simulink model "concept3_simulink_RL"  (R2025a)
settings: Solver=VariableStepAuto  StartTime=0.0  StopTime=Tf  FixedStep=0.001  MaxStep=0.01  MinStep=0.0001  RelTol=1e-3
InitFcn:
  | loaded_data = load('concept3_for_sim.mat');
  | robot = loaded_data.robot;
  | robot.DataFormat = 'column';
values from neighbouring files (symbols this model uses):
  mass = 40    [RL_main.m]    (also in baseline_sim.m)
  obs_vec = opa    [RL_main.m]    (also in baseline_sim.m)
  port = data(n, :)    [RL_main.m]    (also in baseline_sim.m = port_pos_data(n,:))
  port_num = 10    [RL_main.m]    (also in baseline_sim.m)
  port_target = AB2port(port_num)    [RL_main.m]    (also in baseline_sim.m)
  q0arm = rad2deg([-1.283; -1.622; 2.2761853; -1.8021853; 1.112; 1.859; 0.05328])    [RL_main.m]    (also in baseline_sim.m)
  q0b = [1; 0; 0; 0; 0; 0; 0]    [RL_main.m]    (also in baseline_sim.m = [1;0;0;0;0;0;0])
  sat_docked = AB2port(sat_docked_num)    [RL_main.m]    (also in baseline_sim.m)
  sat_docked_num = 6    [RL_main.m]    (also in baseline_sim.m)
  sim_state = 1    [RL_main.m]    (also in baseline_sim.m)
  Tlog = 0.1    [RL_main.m]    (also in baseline_sim.m)
  use_RL = 1    [RL_main.m]    (also in baseline_sim.m)
undefined symbols (not defined in the file or in its folder): opa, target, X, Y, Z
libraries: sm_lib x133, nesl_utility x67, simulink_extras x3, rllib x2
(part 1 of 6)
settings Model: Creator=Junesuk  LastModifiedBy=Junesuk
settings ExplorerConfigSet: InternalSimMechanicsExplorerSettings=|
  | <ExplorerConfiguration>
  | 
  |   <canonicalview>default</canonicalview>
  | 
  |   <TilePanel>
  |     <TileInfo>
  |       <Tiles Columns="1" Count="1" Height="644" Rows="1" Width="984">
  |         <Row Weight="1"/>
  |         <Column Weight="1"/>
  |         <Tile Height="1" Width="1" X="0" Y="0"/>
  |       </Tiles>
  |     </TileInfo>
  |     <SceneInfo>
  |       <SceneViewer>
  |         <IsThisViewStd>
  |           <IsStandardView>off</IsStandardView>
  |           <StandardViewName>Front</StandardViewName>
  |         </IsThisViewStd>
  |         <BGColor>
  |           <R>1</R>
  |           <G>1</G>
  |           <B>1</B>
  |           <A>1</A>
  |         </BGColor>
  |         <Camera>
  |           <DoPerspective>off</DoPerspective>
  |           <Position>
  |             <X>21.646149636080793</X>
  |             <Y>-1.0053245677685836</Y>
  |             <Z>2.2639877275739697</Z>
  |           </Position>
  |           <Center>
  |             <X>0.33501300739641093</X>
  |             <Y>0.083525792263903942</Y>
  |             <Z>0.40625179063450656</Z>
  |           </Center>
  |           <Up>
  |             <X>-0.095945200689781199</X>
  |             <Y>-0.22258518034193089</Y>
  |             <Z>0.97018057904533828</Z>
  |           </Up>
  |           <XLim>2.365123016199409</XLim>
  |           <YLim>2.365123016199409</YLim>
  |           <ViewLimDist>0.01</ViewLimDist>
  |         </Camera>
  |       </SceneViewer>
  |     </SceneInfo>
  |   </TilePanel>
  | 
  |   <MechEditorPanel>
  |     <GfxPanelCameraMap/>
  |     <Cameras/>
  |     <VideoCreator>
  |       <IncludeTiles>All</IncludeTiles>
  |       <IncludeTime>on</IncludeTime>
  |       <IncludeWorldFrame>off</IncludeWorldFrame>
  |       <PlaybackSpeedRatio>1</PlaybackSpeedRatio>
  |       <FrameRate>30</FrameRate>
  |       <FrameSize>auto</FrameSize>
  |       <VideoFormat>UncompressedAVI</VideoFormat>
  |     </VideoCreator>
  |   </MechEditorPanel>
  | 
  |   <PlaybackSettings>
  |     <PlaybackSpeedFactor>16</PlaybackSpeedFactor>
  |   </PlaybackSettings>
  | 
  | </ExplorerConfiguration>

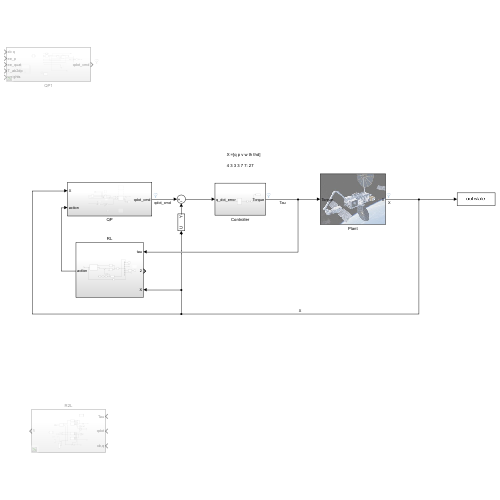
[thumbnail: Simulink's stored preview of the top-level diagram]
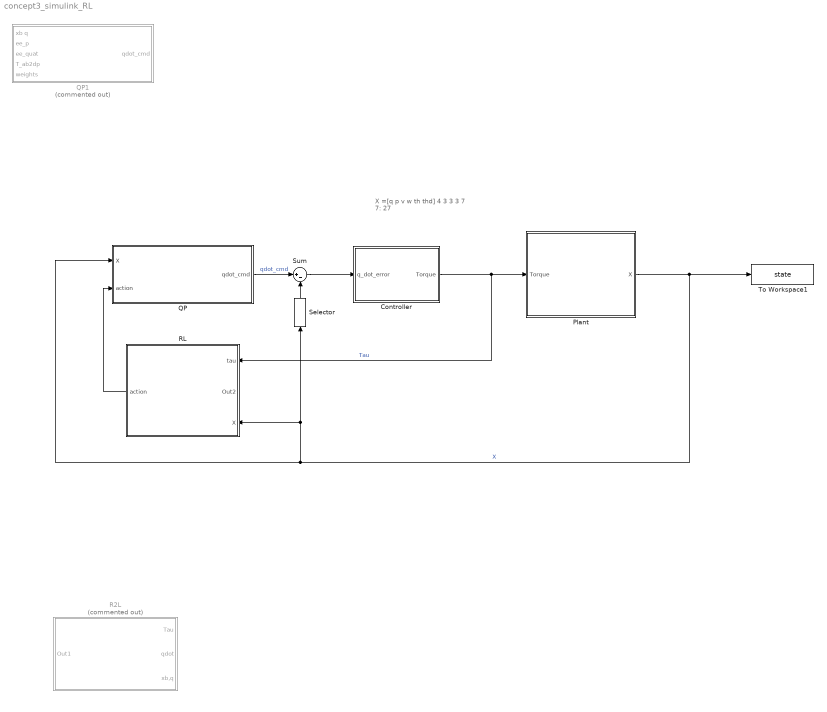
== system concept3_simulink_RL ==
  note: X =[q p v w th thd]
      |
      | 4 3 3 3 7 7: 27
  Controller : Subsystem
  Plant : Subsystem
      mask Display: image('1.jpg');
  QP : Subsystem
  QP1 : Subsystem  Commented=on
  R2L : Subsystem  Commented=on
  RL : Subsystem
      settings: PortSchema="{\"entries\":[{\"content\":{\"sides\":[{\"content\":{\"connectorIds\":[\"In1\",\"Out2\",\"In2\"]},\"type\":\"ConnectorPlacement.EquallySpacedRectSide\",\"uuid\":\"81336b0f-87da-4949-bb3f-96bdd0722e32\"},{\"content\":{\"connectorIds\":[\"Out1\"],\"side\":\"RIGHT\"},\"type\":\"ConnectorPlacement.EquallySpacedRectSide\",\"uuid\":\"5ebe1975-ec97-4e49-ac6a-50b9e3487ed2\"},{\"content\":{\"side\":\"TOP\"},\"type\":\"ConnectorPlacement.EquallySpacedRectSide\",\"uuid\":\"c24f2ad8-8f66-451d-b311-007f5efa803c\"}]},\"type\":\"ConnectorPlacement.EquallySpacedConnector\",\"uuid\":\"e8b94ec5-1840-41b7-8daf-8d62ee1595ef\"}],\"packageUris\":[\"http://schema.mathworks.com/mf0/Connector/R2020b\"],\"version\":\"1.0\"}"
  Selector : Selector  InputPortWidth=27  IndexOptions=Index vector (dialog)  Indices=[21 22 23 24 25 26 27]  OutputSizes=1
  Sum : Sum  Inputs=|+-
  To Workspace1 : ToWorkspace  VariableName=state  SaveFormat=Timeseries  SampleTime=Tlog
  wires:
  Plant/1(X) -> To Workspace1/1, QP/1(X), Selector/1, RL/2(X)  "X"
  Sum/1 -> Controller/1(q_dot_error)
  Controller/1(Torque) -> RL/1(tau), Plant/1(Torque)  "Tau"
  QP/1(qdot_cmd) -> Sum/1  "qdot_cmd"
  RL/1(action) -> QP/2(action)
  Selector/1 -> Sum/2

== system concept3_simulink_RL/Controller ==
  q_dot_error : Inport
  MATLAB Function : MATLAB Function  TreatAsAtomicUnit=on
  Rate Limiter : RateLimiter  RisingSlewLimit=80  FallingSlewLimit=-80  SampleTimeMode=inherited
  Saturation : Saturate  UpperLimit=3  LowerLimit=-3
  To Workspace1 : ToWorkspace  VariableName=torque  SaveFormat=Timeseries  SampleTime=Tlog
  Torque : Outport
  wires:
  Saturation/1 -> To Workspace1/1, Torque/1
  q_dot_error/1 -> MATLAB Function/1(qdot_err)
  MATLAB Function/1(Torque) -> Rate Limiter/1
  Rate Limiter/1 -> Saturation/1

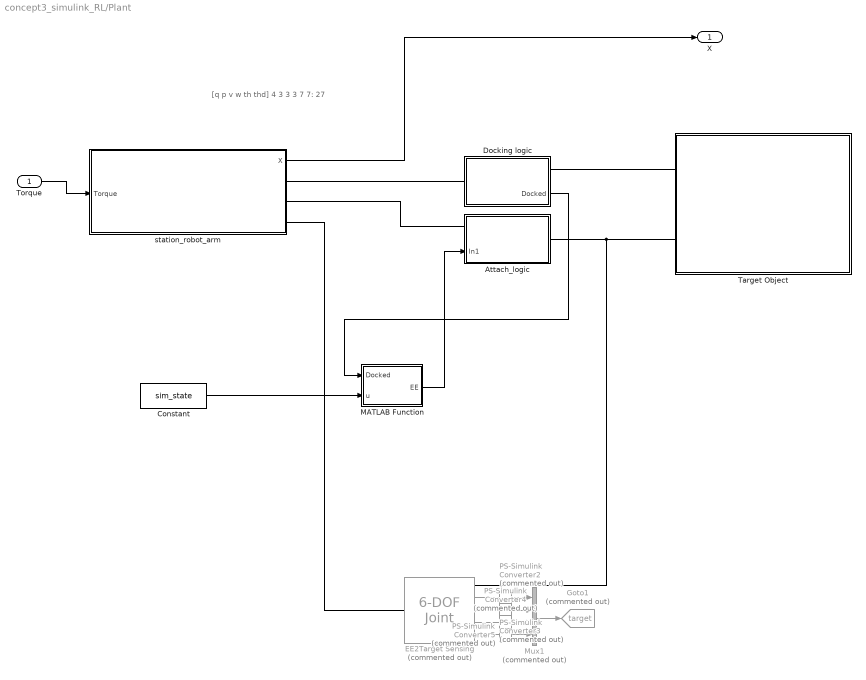
== system concept3_simulink_RL/Plant ==
  note: [q p v w th thd]
      |
      | 4 3 3 3 7 7: 27
  Torque : Inport
  Attach_logic : Subsystem
      settings: PortSchema="{\"entries\":[{\"content\":{\"sides\":[{\"content\":{\"connectorIds\":[\"LConn1\",\"In1\"]},\"type\":\"ConnectorPlacement.EquallySpacedRectSide\",\"uuid\":\"12d0cedd-e218-4f17-9320-f216ac9747ac\"},{\"content\":{\"connectorIds\":[\"RConn1\"],\"side\":\"RIGHT\"},\"type\":\"ConnectorPlacement.EquallySpacedRectSide\",\"uuid\":\"fd28970a-cca5-4053-a7a0-12fc7f529469\"},{\"content\":{\"side\":\"TOP\"},\"type\":\"ConnectorPlacement.EquallySpacedRectSide\",\"uuid\":\"e9d689cc-5bb9-4a0d-a40b-d0a8c8edca38\"}]},\"type\":\"ConnectorPlacement.EquallySpacedConnector\",\"uuid\":\"9791f5c1-0484-4ef0-8b6a-77682d20579a\"}],\"packageUris\":[\"http://schema.mathworks.com/mf0/Connector/R2020b\"],\"version\":\"1.0\"}"
  Constant : Constant  Value=sim_state
  Docking logic : Subsystem
      settings: PortSchema="{\"entries\":[{\"content\":{\"sides\":[{\"content\":{\"connectorIds\":[\"LConn1\"]},\"type\":\"ConnectorPlacement.EquallySpacedRectSide\",\"uuid\":\"76e864fd-fcf6-40cb-8d0c-a293f5f8e793\"},{\"content\":{\"connectorIds\":[\"RConn1\",\"Out1\"],\"side\":\"RIGHT\"},\"type\":\"ConnectorPlacement.EquallySpacedRectSide\",\"uuid\":\"51e0a38e-4dda-40d7-8539-b3b2212d4dbb\"},{\"content\":{\"side\":\"TOP\"},\"type\":\"ConnectorPlacement.EquallySpacedRectSide\",\"uuid\":\"08ea25f5-31f4-4a06-bacf-9e22bf3b7d63\"}]},\"type\":\"ConnectorPlacement.EquallySpacedConnector\",\"uuid\":\"c97bdcdc-89c7-4c9e-882d-350e4fa10246\"}],\"packageUris\":[\"http://schema.mathworks.com/mf0/Connector/R2020b\"],\"version\":\"1.0\"}"
  EE2Target Sensing : sm_lib/Joints/6-DOF Joint  Commented=on  JointMode=Normal  CompositeWrenchDir=FollowerOnBase  CompositeWrenchFrame=BaseFrame  SenseConstraintForce=off  SenseConstraintTorque=off  SenseTotalForce=off  SenseTotalTorque=off  PxPositionTargetSpecify=on  PxPositionTargetPriority=Low  PxPositionTargetValue=target(1)  PxPositionTargetValueUnits=m  PxVelocityTargetSpecify=off  PxVelocityTargetPriority=High  PxVelocityTargetValue=0  PxVelocityTargetValueUnits=m/s  PxEquilibriumPosition=0  PxEquilibriumPositionUnits=m  PxSpringStiffness=0  PxSpringStiffnessUnits=N/m  PxDampingCoefficient=0  PxDampingCoefficientUnits=N/(m/s)  PxLowerLimitSpecify=off  PxLowerLimitBound=-1  PxLowerLimitBoundUnits=m  PxLowerLimitStiffness=1e6  PxLowerLimitStiffnessUnits=N/m  PxLowerLimitDamping=1e3  PxLowerLimitDampingUnits=N/(m/s)  PxLowerLimitTransitionRegionWidth=1e-4  PxLowerLimitTransitionRegionWidthUnits=m  PxUpperLimitSpecify=off  PxUpperLimitBound=1  PxUpperLimitBoundUnits=m  PxUpperLimitStiffness=1e6  PxUpperLimitStiffnessUnits=N/m  PxUpperLimitDamping=1e3  PxUpperLimitDampingUnits=N/(m/s)  PxUpperLimitTransitionRegionWidth=1e-4  PxUpperLimitTransitionRegionWidthUnits=m  PxTorqueActuationMode=NoTorque  PxMotionActuationMode=ComputedMotion  PxSensePosition=on  PxSenseVelocity=off  PxSenseAcceleration=off  PxSenseTorqueForce=off  PxSenseLowerLimitTorqueForce=off  PxSenseUpperLimitTorqueForce=off  PyPositionTargetSpecify=on  PyPositionTargetPriority=Low  PyPositionTargetValue=target(2)  PyPositionTargetValueUnits=m  PyVelocityTargetSpecify=off  PyVelocityTargetPriority=High  PyVelocityTargetValue=0  PyVelocityTargetValueUnits=m/s  PyEquilibriumPosition=0  PyEquilibriumPositionUnits=m  PySpringStiffness=0  PySpringStiffnessUnits=N/m  PyDampingCoefficient=0  PyDampingCoefficientUnits=N/(m/s)  PyLowerLimitSpecify=off  PyLowerLimitBound=-1  PyLowerLimitBoundUnits=m  PyLowerLimitStiffness=1e6  PyLowerLimitStiffnessUnits=N/m  PyLowerLimitDamping=1e3  PyLowerLimitDampingUnits=N/(m/s)  PyLowerLimitTransitionRegionWidth=1e-4  PyLowerLimitTransitionRegionWidthUnits=m  PyUpperLimitSpecify=off  PyUpperLimitBound=1  PyUpperLimitBoundUnits=m  PyUpperLimitStiffness=1e6  PyUpperLimitStiffnessUnits=N/m  PyUpperLimitDamping=1e3  PyUpperLimitDampingUnits=N/(m/s)  PyUpperLimitTransitionRegionWidth=1e-4  PyUpperLimitTransitionRegionWidthUnits=m  PyTorqueActuationMode=NoTorque  PyMotionActuationMode=ComputedMotion  PySensePosition=on  PySenseVelocity=off  PySenseAcceleration=off  PySenseTorqueForce=off  PySenseLowerLimitTorqueForce=off  PySenseUpperLimitTorqueForce=off  PzPositionTargetSpecify=on  PzPositionTargetPriority=Low  PzPositionTargetValue=target(3)  PzPositionTargetValueUnits=m  PzVelocityTargetSpecify=off  PzVelocityTargetPriority=High  PzVelocityTargetValue=0  PzVelocityTargetValueUnits=m/s  PzEquilibriumPosition=0  PzEquilibriumPositionUnits=m  PzSpringStiffness=0  PzSpringStiffnessUnits=N/m  PzDampingCoefficient=0  PzDampingCoefficientUnits=N/(m/s)  PzLowerLimitSpecify=off  PzLowerLimitBound=-1  PzLowerLimitBoundUnits=m  PzLowerLimitStiffness=1e6  PzLowerLimitStiffnessUnits=N/m  PzLowerLimitDamping=1e3  PzLowerLimitDampingUnits=N/(m/s)  PzLowerLimitTransitionRegionWidth=1e-4  PzLowerLimitTransitionRegionWidthUnits=m  PzUpperLimitSpecify=off  PzUpperLimitBound=1  PzUpperLimitBoundUnits=m  PzUpperLimitStiffness=1e6  PzUpperLimitStiffnessUnits=N/m  PzUpperLimitDamping=1e3  PzUpperLimitDampingUnits=N/(m/s)  PzUpperLimitTransitionRegionWidth=1e-4  PzUpperLimitTransitionRegionWidthUnits=m  PzTorqueActuationMode=NoTorque  PzMotionActuationMode=ComputedMotion  PzSensePosition=on  PzSenseVelocity=off  PzSenseAcceleration=off  PzSenseTorqueForce=off  PzSenseLowerLimitTorqueForce=off  PzSenseUpperLimitTorqueForce=off  SphPositionTargetSpecify=on  SphPositionTargetPriority=Low  SphPositionTargetRotationMethod=RotationSequence  SphPositionTargetFollAlignAxisA=+X  SphPositionTargetBaseAlignAxisA=+Y  SphPositionTargetFollAlignAxisB=+Y  SphPositionTargetBaseAlignAxisB=+Z  SphPositionTargetRotationStandardAxis=+Z  SphPositionTargetRotationAngle=0  SphPositionTargetRotationAngleUnits=deg  SphPositionTargetRotationArbitraryAxis=[0 0 1]  SphPositionTargetRotationSequenceAxes=FollowerAxes  SphPositionTargetRotationSequence=ZYX  SphPositionTargetRotationSequenceAngles=[target(4) target(5) target(6) ]  SphPositionTargetRotationSequenceAnglesUnits=deg  SphPositionTargetRotationMatrix=[1 0 0;0 1 0;0 0 1]  SphPositionTargetQuaternion=[1 0 0 0]  SphVelocityTargetSpecify=off  SphVelocityTargetPriority=High  SphVelocityTargetValue=[0 0 0]  SphVelocityTargetValueUnits=deg/s  SphVelocityTargetInFollowerFrame=on  SphEqPosRotationMethod=None  SphEqPosFollAlignAxisA=+X  SphEqPosBaseAlignAxisA=+Y  SphEqPosFollAlignAxisB=+Y  SphEqPosBaseAlignAxisB=+Z  SphEqPosRotationStandardAxis=+Z  SphEqPosRotationAngle=0  SphEqPosRotationAngleUnits=deg  SphEqPosRotationArbitraryAxis=[0 0 1]  SphEqPosRotationSequenceAxes=FollowerAxes  SphEqPosRotationSequence=XYX  SphEqPosRotationSequenceAngles=[0 0 0]  SphEqPosRotationSequenceAnglesUnits=deg  SphEqPosRotationMatrix=[1 0 0;0 1 0;0 0 1]  SphEqPosQuaternion=[1 0 0 0]  SphSpringStiffness=0  SphSpringStiffnessUnits=N*m/deg  SphDampingCoefficient=0  SphDampingCoefficientUnits=N*m/(deg/s)  SphLowerLimitSpecify=off  SphLowerLimitBound=15  SphLowerLimitBoundUnits=deg  SphLowerLimitStiffness=1e4  SphLowerLimitStiffnessUnits=N*m/deg  SphLowerLimitDamping=10  SphLowerLimitDampingUnits=N*m/(deg/s)  SphLowerLimitTransitionRegionWidth=0.1  SphLowerLimitTransitionRegionWidthUnits=deg  SphUpperLimitSpecify=off  SphUpperLimitBound=45  SphUpperLimitBoundUnits=deg  SphUpperLimitStiffness=1e4  SphUpperLimitStiffnessUnits=N*m/deg  SphUpperLimitDamping=10  SphUpperLimitDampingUnits=N*m/(deg/s)  SphUpperLimitTransitionRegionWidth=0.1  SphUpperLimitTransitionRegionWidthUnits=deg  SphTorqueActuationMode=NoTorque  SphActuateTorqueX=off  SphActuateTorqueY=off  SphActuateTorqueZ=off  SphActuateTorque=off  SphActuationFrame=BaseFrame  SphSensePosition=on  SphSenseVelocityX=off  SphSenseVelocityY=off  SphSenseVelocityZ=off  SphSenseVelocity=off  SphSenseAccelerationX=off  SphSenseAccelerationY=off  SphSenseAccelerationZ=off  SphSenseAcceleration=off  SphSenseLowerLimitTorqueMag=off  SphSenseUpperLimitTorqueMag=off  SphSensingFrame=BaseFrame
  Goto1 : Goto  Commented=on  GotoTag=target  TagVisibility=global
  MATLAB Function : MATLAB Function  TreatAsAtomicUnit=on
  Mux1 : Mux  Commented=on
  PS-Simulink Converter{2..5} (4 alike) : nesl_utility/PS-Simulink Converter  Commented=on  PhysicalDomain=network_engine_domain  SubClassName=ps_output  LeftPortType=input  RightPortType=output  PseudoPeriodic=off  Frequencies=[]  VectorFormat=inherit  Unit=inherit  AffineConversion=off
  Target Object : Subsystem
      mask Display: image('2.jpg');
  station_robot_arm : Subsystem
  X : Outport
  wires:
  Torque/1 -> station_robot_arm/1(Torque)
  station_robot_arm/1(X) -> X/1
  PS-Simulink Converter2/1 -> Mux1/1
  PS-Simulink Converter3/1 -> Mux1/2
  PS-Simulink Converter4/1 -> Mux1/3
  PS-Simulink Converter5/1 -> Mux1/4
  Mux1/1 -> Goto1/1
  Constant/1 -> MATLAB Function/2(u)
  MATLAB Function/1(EE) -> Attach_logic/1(In1)
  Docking logic/1(Docked) -> MATLAB Function/1(Docked)
  connections:
  Target Object/LConn1 -- Docking logic/RConn1
  Attach_logic/RConn1 -- EE2Target Sensing/RConn1 -- Target Object/LConn2
  station_robot_arm/RConn3 -- EE2Target Sensing/LConn1
  station_robot_arm/RConn2 -- Attach_logic/LConn1
  station_robot_arm/RConn1 -- Docking logic/LConn1
  PS-Simulink Converter4/LConn1 -- EE2Target Sensing/RConn4
  EE2Target Sensing/RConn3 -- PS-Simulink Converter3/LConn1
  EE2Target Sensing/RConn2 -- PS-Simulink Converter2/LConn1
  PS-Simulink Converter5/LConn1 -- EE2Target Sensing/RConn5

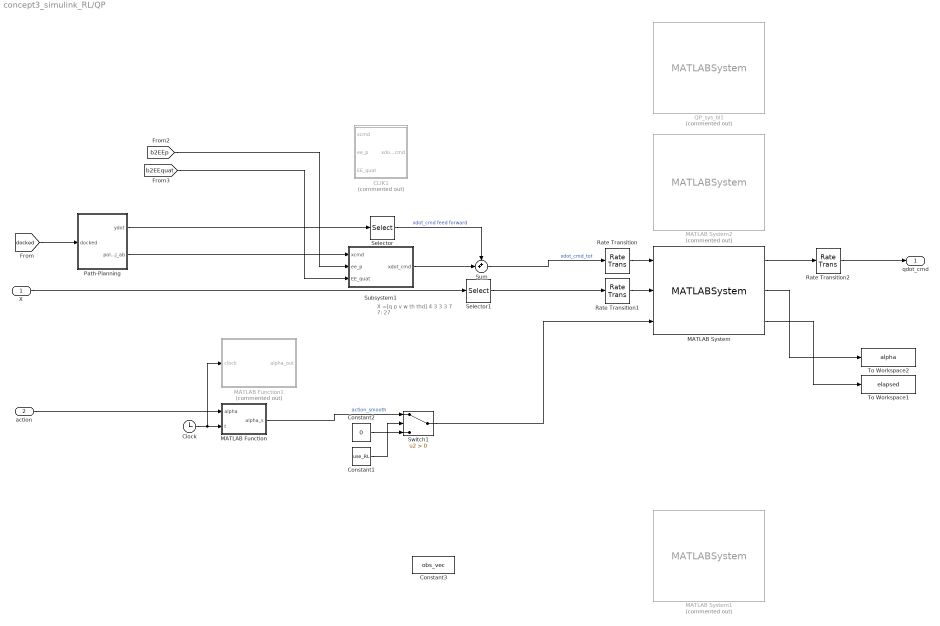
== system concept3_simulink_RL/QP ==
  note: X =[q p v w th thd]
      |
      | 4 3 3 3 7 7: 27
  X : Inport
  action : Inport  Port=2
  CLIK1 : Subsystem  Commented=on
  Clock : Clock
  Constant1 : Constant  Value=use_RL
  Constant2 : Constant  Value=0
  Constant3 : Constant  Value=obs_vec
  MATLAB Function : MATLAB Function  TreatAsAtomicUnit=on
  MATLAB Function1 : MATLAB Function  Commented=on  TreatAsAtomicUnit=on
  MATLAB System : MATLABSystem  System=QP_sys_RL  SimulateUsing=Interpreted execution
      mask Type: QP_sys_RL
  MATLAB System1 : MATLABSystem  Commented=on  System=RH_QP_sys_bl  H_hor=10  lambda_s=0.05  lambda_t=0.1  kp_base=10  SimulateUsing=Interpreted execution
      mask Type: RH_QP_sys_bl
  MATLAB System2 : MATLABSystem  Commented=on  System=Pseudo_inv_sys_RL  SimulateUsing=Interpreted execution
      mask Type: Pseudo_inv_sys_RL
  "Path-Planning " : Subsystem
  QP_sys_bl1 : MATLABSystem  Commented=on  System=QP_sys_bl  null_method=a  kp_base=1  SimulateUsing=Interpreted execution
      mask Type: QP_sys_bl
  Rate Transition : RateTransition  OutPortSampleTime=Tq
  Rate Transition1 : RateTransition  OutPortSampleTime=Tq
  Rate Transition2 : RateTransition
  Selector : Selector  InputPortWidth=6  IndexOptions=Index vector (dialog)  Indices=[4 5 6 1 2 3]  OutputSizes=1
  Selector1 : Selector  InputPortWidth=27  IndexOptions=Index vector (dialog)  Indices=[1 2 3 4 5 6 7 14 15 16 17 18 19 20]  OutputSizes=1
  Subsystem1 : Subsystem
  Sum : Sum  Inputs=++|
  Switch1 : Switch  Criteria=u2 > Threshold  SaturateOnIntegerOverflow=off  InputSameDT=off
  To Workspace1 : ToWorkspace  VariableName=elapsed  SaveFormat=Timeseries  SampleTime=Tlog
  To Workspace2 : ToWorkspace  VariableName=alpha  SaveFormat=Timeseries  SampleTime=Tlog
  qdot_cmd : Outport
  wires:
  [docked] -> "Path-Planning "/1(docked)
  "Path-Planning "/1(ydot) -> Selector/1
  "Path-Planning "/2(poly_traj_ab) -> Subsystem1/1(xcmd)
  Subsystem1/1(xdot_cmd) -> Sum/2
  [b2EEp] -> Subsystem1/2(ee_p)
  [b2EEquat] -> Subsystem1/3(EE_quat)
  Sum/1 -> Rate Transition/1  "xdot_cmd_tot"
  Clock/1 -> MATLAB Function1/1(clock), MATLAB Function/2(t)
  Constant2/1 -> Switch1/3
  MATLAB Function/1(alpha_s) -> Switch1/1  "action_smooth"
  X/1 -> Selector1/1
  Selector1/1 -> Rate Transition1/1
  Rate Transition/1 -> MATLAB System/1
  Rate Transition2/1 -> qdot_cmd/1
  Constant1/1 -> Switch1/2
  action/1 -> MATLAB Function/1(alpha)
  Selector/1 -> Sum/1  "xdot_cmd feed forward"
  MATLAB System/1 -> Rate Transition2/1
  MATLAB System/3 -> To Workspace1/1
  Rate Transition1/1 -> MATLAB System/2
  MATLAB System/2 -> To Workspace2/1
  Switch1/1 -> MATLAB System/3

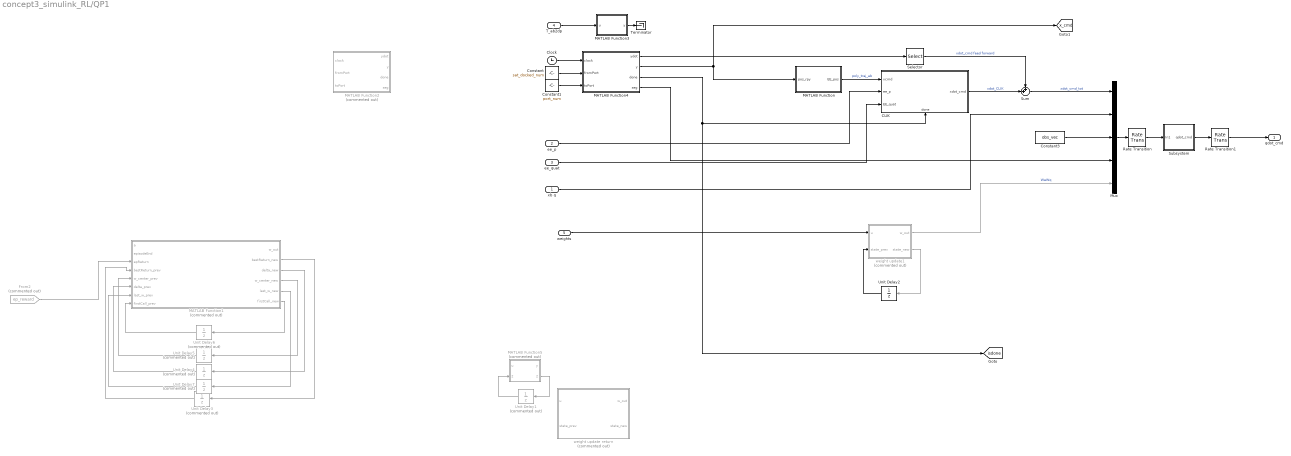
== system concept3_simulink_RL/QP1 ==
  xb q : Inport
  ee_p : Inport  Port=2
  ee_quat : Inport  Port=3
  T_ab2dp : Inport  Port=4
  weights : Inport  Port=5
  CLIK : Subsystem
      settings: PortSchema="{\"entries\":[{\"content\":{\"sides\":[{\"content\":{\"connectorIds\":[\"In1\",\"In2\",\"In3\"]},\"type\":\"ConnectorPlacement.EquallySpacedRectSide\",\"uuid\":\"53537e45-b349-4ff7-b811-6fdcc057d7d2\"},{\"content\":{\"connectorIds\":[\"Out1\"],\"side\":\"RIGHT\"},\"type\":\"ConnectorPlacement.EquallySpacedRectSide\",\"uuid\":\"c6f0bded-37ff-429d-8334-4fbe19a63c08\"},{\"content\":{\"side\":\"TOP\"},\"type\":\"ConnectorPlacement.EquallySpacedRectSide\",\"uuid\":\"dac46d9f-48be-42ca-88ab-9eef949b6b0e\"},{\"content\":{\"connectorIds\":[\"In4\"],\"side\":\"BOTTOM\"},\"type\":\"ConnectorPlacement.EquallySpacedRectSide\",\"uuid\":\"26bd092c-8c32-427f-a0d8-6b9ca2752a43\"}]},\"type\":\"ConnectorPlacement.EquallySpacedConnector\",\"uuid\":\"0be7ea49-038f-4080-8c33-dbecb36af2ab\"}],\"packageUris\":[\"http://schema.mathworks.com/mf0/Connector/R2020b\"],\"version\":\"1.0\"}"
  Clock : Clock
  Constant : Constant  Value=sat_docked_num
  Constant1 : Constant  Value=port_num
  Constant3 : Constant  Value=obs_vec
  From2 : From  Commented=on  GotoTag=ep_reward  TagVisibility=global
  MATLAB Function : MATLAB Function  TreatAsAtomicUnit=on
  MATLAB Function1 : MATLAB Function  Commented=on  TreatAsAtomicUnit=on
  MATLAB Function2 : MATLAB Function  Commented=on  TreatAsAtomicUnit=on
  MATLAB Function3 : MATLAB Function  TreatAsAtomicUnit=on
  MATLAB Function4 : MATLAB Function  TreatAsAtomicUnit=on
  MATLAB Function5 : MATLAB Function  Commented=on  TreatAsAtomicUnit=on
  Mux : Mux  Inputs=5
  Rate Transition : RateTransition  OutPortSampleTime=0.1
  Rate Transition1 : RateTransition
  Selector : Selector  InputPortWidth=6  IndexOptions=Index vector (dialog)  Indices=[4 5 6 1 2 3]  OutputSizes=1
  Subsystem : Subsystem
  Sum : Sum  Inputs=++|
  Terminator : Terminator
  Unit Delay{1,3..7} (6 alike) : UnitDelay  Commented=on  SampleTime=-1  HasFrameUpgradeWarning=on
  Unit Delay2 : UnitDelay  SampleTime=-1  HasFrameUpgradeWarning=on
  weight update return : MATLAB Function  Commented=on  TreatAsAtomicUnit=on
  weight update1 : MATLAB Function  Commented=on  TreatAsAtomicUnit=on
  qdot_cmd : Outport
  tag scope: isdone=global, x_cmd=global
  wires:
  MATLAB Function4/3(done) -> CLIK/4(done), [isdone]
  MATLAB Function3/1(y) -> Terminator/1
  Unit Delay6/1 -> MATLAB Function1/8(firstCall_prev)
  MATLAB Function1/6(firstCall_new) -> Unit Delay6/1
  Unit Delay7/1 -> MATLAB Function1/7(last_w_prev)
  MATLAB Function1/5(last_w_new) -> Unit Delay7/1
  Unit Delay4/1 -> MATLAB Function1/6(delta_prev)
  MATLAB Function1/3(delta_new) -> Unit Delay4/1
  Unit Delay5/1 -> MATLAB Function1/5(w_center_prev)
  MATLAB Function1/4(w_center_new) -> Unit Delay5/1
  Unit Delay3/1 -> MATLAB Function1/4(bestReturn_prev)
  MATLAB Function1/2(bestReturn_new) -> Unit Delay3/1
  weights/1 -> weight update1/1(u)
  Unit Delay2/1 -> weight update1/2(state_prev)
  weight update1/2(state_new) -> Unit Delay2/1
  From2/1 -> MATLAB Function1/3(epReturn)
  weight update1/1(w_out) -> Mux/5  "WeWq"
  Unit Delay1/1 -> MATLAB Function5/2(w_prev)
  MATLAB Function5/2(w_new) -> Unit Delay1/1
  Rate Transition1/1 -> qdot_cmd/1
  Rate Transition/1 -> Subsystem/1(In1)
  Mux/1 -> Rate Transition/1
  Subsystem/1(qdot_cmd) -> Rate Transition1/1
  MATLAB Function4/4(seg) -> Mux/4
  CLIK/1(xdot_cmd) -> Sum/2  "xdot_CLIK"
  Constant3/1 -> Mux/3
  T_ab2dp/1 -> MATLAB Function3/1(u)
  MATLAB Function4/2(y) -> MATLAB Function/1(pos_rpy), [x_cmd]
  MATLAB Function4/1(ydot) -> Selector/1
  Selector/1 -> Sum/1  "xdot_cmd feed forward"
  Sum/1 -> Mux/1  "xdot_cmd_tot"
  MATLAB Function/1(EE_pos) -> CLIK/1(xcmd)  "poly_traj_ab"
  ee_quat/1 -> CLIK/3(EE_quat)
  ee_p/1 -> CLIK/2(ee_p)
  Constant1/1 -> MATLAB Function4/3(toPort)
  Constant/1 -> MATLAB Function4/2(fromPort)
  Clock/1 -> MATLAB Function4/1(clock)
  xb q/1 -> Mux/2

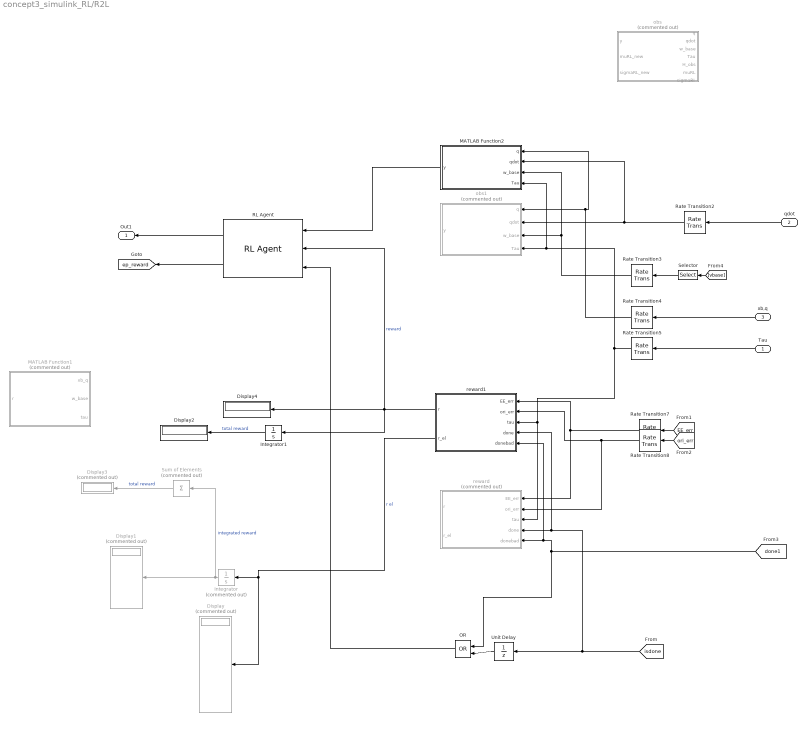
== system concept3_simulink_RL/R2L ==
  Tau : Inport
  qdot : Inport  Port=2
  xb,q : Inport  Port=3
  Display : Display  Commented=on
  Display1 : Display  Commented=on
  Display2 : Display
  Display3 : Display  Commented=on
  Display4 : Display
  Integrator : Integrator  Commented=on
  Integrator1 : Integrator
  MATLAB Function1 : MATLAB Function  Commented=on  TreatAsAtomicUnit=on
  MATLAB Function2 : MATLAB Function  TreatAsAtomicUnit=on
  OR : Logic  Operator=OR  IconShape=distinctive  AllPortsSameDT=off  OutDataTypeStr=boolean
  RL Agent : rllib/RL Agent  Agent=agent  ExternalActionAsInput=off  ProvideLastAction=off  ProvideCumRwd=on  TreatAsDirectFeedthrough=on  UseStrictObservationDataTypes=off
  Rate Transition{2..5,7..8} (6 alike) : RateTransition  OutPortSampleTime=Ts
  Selector : Selector  InputPortWidth=6  IndexOptions=Index vector (dialog)  Indices=[4 5 6]  OutputSizes=1
  Sum of Elements : Sum  Commented=on  Inputs=+
  Unit Delay : UnitDelay  SampleTime=-1  HasFrameUpgradeWarning=on
  obs : MATLAB Function  Commented=on  TreatAsAtomicUnit=on
  obs1 : MATLAB Function  Commented=on  TreatAsAtomicUnit=on
  reward : MATLAB Function  Commented=on  TreatAsAtomicUnit=on
  reward1 : MATLAB Function  TreatAsAtomicUnit=on
  Out1 : Outport
  tag scope: ep_reward=global
  wires:
  [vbase] -> Selector/1
  Selector/1 -> Rate Transition3/1
  qdot/1 -> Rate Transition2/1
  xb,q/1 -> Rate Transition4/1
  RL Agent/1 -> Out1/1
  Integrator/1 -> Display1/1, Sum of Elements/1  "integrated reward"
  Sum of Elements/1 -> Display3/1  "total reward"
  Integrator1/1 -> Display2/1  "total reward"
  Rate Transition5/1 -> reward/3(tau), reward1/3(tau), MATLAB Function2/4(Tau), obs1/4(Tau)
  Rate Transition2/1 -> obs1/2(qdot), MATLAB Function2/2(qdot)
  Tau/1 -> Rate Transition5/1
  Rate Transition4/1 -> obs1/1(q), MATLAB Function2/1(q)
  Rate Transition3/1 -> MATLAB Function2/3(w_base), obs1/3(w_base)
  RL Agent/2 -> [ep_reward]
  [ori_err] -> Rate Transition8/1
  [EE_err] -> Rate Transition7/1
  Rate Transition7/1 -> reward1/1(EE_err), reward/1(EE_err)
  Rate Transition8/1 -> reward1/2(ori_err), reward/2(ori_err)
  [isdone] -> reward1/4(done), reward/4(done), Unit Delay/1
  [done1] -> OR/1, reward1/5(donebad), reward/5(donebad)
  Unit Delay/1 -> OR/2
  OR/1 -> RL Agent/3
  reward1/2(r_el) -> Display/1, Integrator/1  "r el"
  reward1/1(r) -> Integrator1/1, RL Agent/2, Display4/1  "reward"
  MATLAB Function2/1(y) -> RL Agent/1

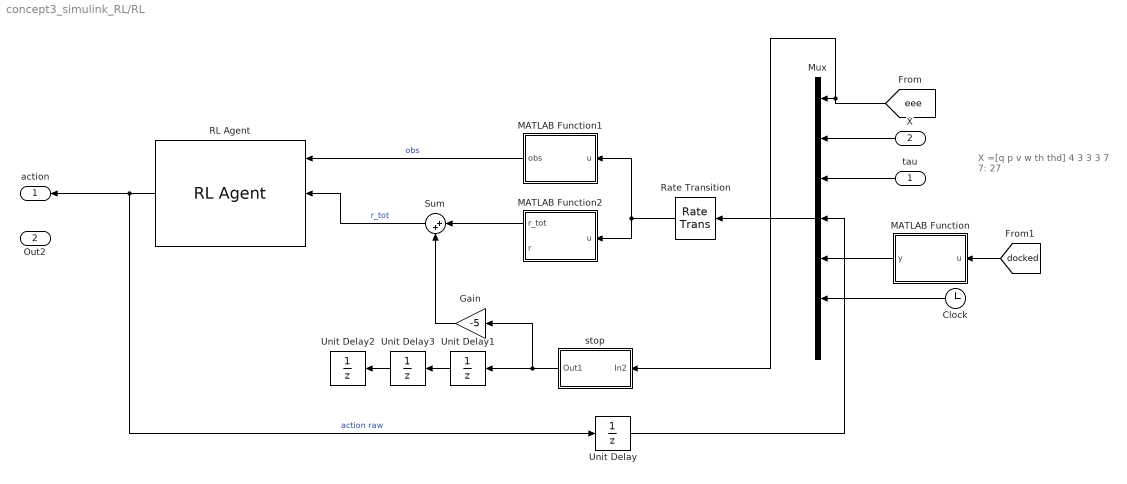
== system concept3_simulink_RL/RL ==
  note: X =[q p v w th thd]
      |
      | 4 3 3 3 7 7: 27
  tau : Inport
  X : Inport  Port=2
  Clock : Clock
  Gain : Gain  Gain=-5
  MATLAB Function : MATLAB Function  TreatAsAtomicUnit=on
  MATLAB Function1 : MATLAB Function  TreatAsAtomicUnit=on
  MATLAB Function2 : MATLAB Function  TreatAsAtomicUnit=on
  Mux : Mux  Inputs=7
  RL Agent : rllib/RL Agent  Agent=agent  ExternalActionAsInput=off  ProvideLastAction=off  ProvideCumRwd=off  TreatAsDirectFeedthrough=on  UseStrictObservationDataTypes=off
  Rate Transition : RateTransition  OutPortSampleTime=T_RL
  Sum : Sum  Inputs=|++
  Unit Delay{,1..3} (4 alike) : UnitDelay  SampleTime=-1  HasFrameUpgradeWarning=on
  stop : Subsystem
  action : Outport
  Out2 : Outport  Port=2
  wires:
  X/1 -> Mux/2
  [eee] -> stop/1(In2), Mux/1
  tau/1 -> Mux/3
  RL Agent/1 -> action/1, Unit Delay/1  "action raw"
  Unit Delay/1 -> Mux/4
  Rate Transition/1 -> MATLAB Function1/1(u), MATLAB Function2/1(u)
  Mux/1 -> Rate Transition/1
  Sum/1 -> RL Agent/2  "r_tot"
  MATLAB Function1/1(obs) -> RL Agent/1  "obs"
  stop/1(Out1) -> Gain/1, Unit Delay1/1
  MATLAB Function2/1(r_tot) -> Sum/1
  [docked] -> MATLAB Function/1(u)
  MATLAB Function/1(y) -> Mux/5
  Clock/1 -> Mux/6
  Unit Delay1/1 -> Unit Delay3/1
  Unit Delay3/1 -> Unit Delay2/1
  Gain/1 -> Sum/2

== system concept3_simulink_RL/Plant/Attach_logic ==
  note: -1이 해제, 0이 연결
  In1 : Inport
  Attach : Display
  Attach sensor : Subsystem  Commented=on
  Constant : Constant  Value=-1
  Constant1 : Constant  Value=0
  Simulink-PS Converter : nesl_utility/Simulink-PS Converter  PhysicalDomain=network_engine_domain  SubClassName=ps_input  LeftPortType=input  RightPortType=output  PseudoPeriodic=off  Frequencies=[]  NoiseDistribution=none  NoiseParameters=[]  Unit=1  AffineConversion=off  FilteringAndDerivatives=provide  SimscapeFilterOrder=1  InputFilterTimeConstant=0.001  UdotUserProvided=0
  Switch : Switch  Criteria=u2 > Threshold  SaturateOnIntegerOverflow=off  InputSameDT=off
  Unit Delay : UnitDelay  SampleTime=-1  HasFrameUpgradeWarning=on
  Weld Joint : sm_lib/Joints/Weld Joint  JointMode=ProvidedByInput  CompositeWrenchDir=FollowerOnBase  CompositeWrenchFrame=BaseFrame  SenseConstraintForce=off  SenseConstraintTorque=off  SenseTotalForce=off  SenseTotalTorque=off
  EE : PMIOPort  Side=Left
  Sat : PMIOPort  Port=2  Side=Right
  tag scope: attach=global
  wires:
  Attach sensor/1(attach) -> Attach/1, Unit Delay/1, [attach]
  Constant/1 -> Switch/3
  Switch/1 -> Simulink-PS Converter/1
  Constant1/1 -> Switch/1
  In1/1 -> Switch/2
  connections:
  EE/RConn1 -- Attach sensor/LConn1 -- Weld Joint/LConn1
  Weld Joint/RConn1 -- Attach sensor/RConn1 -- Sat/RConn1
  Simulink-PS Converter/RConn1 -- Weld Joint/LConn2

== system concept3_simulink_RL/Plant/Docking logic ==
  note: -1이 해제, 0이 연결
  Constant : Constant  Value=-1
  Constant1 : Constant  Value=0
  Docked disp : Display
  Docking sensor : Subsystem
  Simulink-PS Converter : nesl_utility/Simulink-PS Converter  PhysicalDomain=network_engine_domain  SubClassName=ps_input  LeftPortType=input  RightPortType=output  PseudoPeriodic=off  Frequencies=[]  NoiseDistribution=none  NoiseParameters=[]  Unit=1  AffineConversion=off  FilteringAndDerivatives=provide  SimscapeFilterOrder=1  InputFilterTimeConstant=0.001  UdotUserProvided=0
  Switch : Switch  Criteria=u2 > Threshold  SaturateOnIntegerOverflow=off  InputSameDT=off
  Unit Delay : UnitDelay  SampleTime=-1  HasFrameUpgradeWarning=on
  Weld Joint : sm_lib/Joints/Weld Joint  JointMode=ProvidedByInput  CompositeWrenchDir=FollowerOnBase  CompositeWrenchFrame=BaseFrame  SenseConstraintForce=off  SenseConstraintTorque=off  SenseTotalForce=off  SenseTotalTorque=off
  Port1 : PMIOPort  Side=Left
  Sat : PMIOPort  Port=2  Side=Right
  Docked : Outport
  tag scope: docked=global
  wires:
  Docking sensor/1(Dock) -> Unit Delay/1, Docked disp/1
  Constant/1 -> Switch/3
  Switch/1 -> Simulink-PS Converter/1
  Constant1/1 -> Switch/1
  Unit Delay/1 -> Docked/1, [docked], Switch/2
  connections:
  Sat/RConn1 -- Weld Joint/RConn1 -- Docking sensor/RConn1
  Weld Joint/LConn1 -- Port1/RConn1 -- Docking sensor/LConn1
  Simulink-PS Converter/RConn1 -- Weld Joint/LConn2

== system concept3_simulink_RL/Plant/Target Object ==
  Brick Solid1 : sm_lib/Body Elements/Brick Solid  BrickDimensions=[0.4 0.4 0.5]  BrickDimensionsUnits=m  ExportEntireGeometry=off  InertiaType=CalculateFromGeometry  BasedOnType=Mass  Density=1000  DensityUnits=kg/m^3  Mass=40  MassUnits=kg  CenterOfMass=[0 0 0]  CenterOfMassUnits=m  MomentsOfInertia=[1 1 1]  MomentsOfInertiaUnits=kg*m^2  ProductsOfInertia=[0 0 0]  ProductsOfInertiaUnits=kg*m^2  GraphicType=FromGeometry  MarkerShape=Cube  MarkerSize=10  GraphicVisPropType=SimpleVisualProperties  GraphicDiffuseColor=[0.5 0.5 0.5]  GraphicOpacity=0  GraphicSpecularColor=[0.5 0.5 0.5 1.0]  GraphicAmbientColor=[0.15 0.15 0.15 1.0]  GraphicEmissiveColor=[0.0 0.0 0.0 1.0]  GraphicShininess=75  DoExposeReferenceFrame=on  SerializedFrames=<Frames><Frame><Id>Frame1</Id><Value><Name>F1</Name><Origin><Source>GeometricFeature</Source><FeatureName>-z surface</FeatureName></Origin><PrimaryAxis><DefinedDirection>+Z</DefinedDirection><Source>ReferenceFrame</Source><SourceDirection>+Z</SourceDirection><FeatureName></FeatureName></PrimaryAxis><SecondaryAxis><DefinedDirection>+X</DefinedDirection><Source>ReferenceFrame</Source><SourceDirection>+X</SourceDirection><FeatureName></FeatureName></SecondaryAxis></Value></Frame></Frames>
  File Solid : sm_lib/Body Elements/File Solid  ExtGeomFileName=meshes\module.stl  UnitType=Custom  ExtGeomFileUnits=mm  StepReaderType=HEX  ExportConvexHullGeometry=off  InertiaType=CalculateFromGeometry  BasedOnType=Mass  Density=1000  DensityUnits=kg/m^3  Mass=0  MassUnits=kg  CenterOfMass=[0 0 0]  CenterOfMassUnits=m  MomentsOfInertia=[1 1 1]  MomentsOfInertiaUnits=kg*m^2  ProductsOfInertia=[0 0 0]  ProductsOfInertiaUnits=kg*m^2  GraphicType=FromGeometry  MarkerShape=Sphere  MarkerSize=10  GraphicVisPropType=SimpleVisualProperties  GraphicDiffuseColor=[1 0.6667 0]  GraphicOpacity=1  GraphicSpecularColor=[0.5 0.5 0.5 1.0]  GraphicAmbientColor=[0.15 0.15 0.15 1.0]  GraphicEmissiveColor=[0.0 0.0 0.0 1.0]  GraphicShininess=75  DoExposeReferenceFrame=on  SerializedFrames=<Frames/>
  d2 : sm_lib/Frames and Transforms/Rigid Transform  RotationMethod=StandardAxis  FollAlignAxisA=+X  BaseAlignAxisA=+Y  FollAlignAxisB=+Y  BaseAlignAxisB=+Z  RotationStandardAxis=+X  RotationAngle=180  RotationAngleUnits=deg  RotationArbitraryAxis=[0 0 1]  RotationSequenceAxes=FollowerAxes  RotationSequence=XYX  RotationSequenceAngles=[0 0 0]  RotationSequenceAnglesUnits=deg  RotationMatrix=[1 0 0;0 1 0;0 0 1]  Quaternion=[1 0 0 0]  TranslationMethod=Cartesian  TranslationCartesianOffset=[0 0 0.505 ]  TranslationCartesianOffsetUnits=m  TranslationStandardAxis=+Z  TranslationStandardOffset=0  TranslationStandardOffsetUnits=m  TranslationROffset=0  TranslationROffsetUnits=m  TranslationThetaOffset=0  TranslationThetaOffsetUnits=deg  TranslationZOffset=0  TranslationZOffsetUnits=m
  Station attachment point : PMIOPort  Side=Left
  Target attachment point : PMIOPort  Port=2  Side=Left
  connections:
  Target attachment point/RConn1 -- d2/LConn1
  File Solid/RConn1 -- Brick Solid1/LConn1 -- Station attachment point/RConn1 -- d2/RConn1
